simulink model "dtm"  (R2012b)
settings: Solver=ode45  StartTime=0.0  StopTime=15  RelTol=1e-3
settings Model: Creator=eechris  LastModifiedBy=eechris

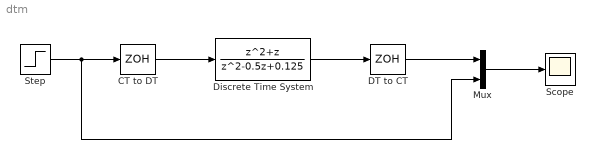
== system dtm ==
  CT to DT : ZeroOrderHold
  DT to CT : ZeroOrderHold
  Discrete Time System : DiscreteTransferFcn  Numerator=[1 1 0]  Denominator=[1 -0.5 0.125]
  Mux : Mux  Inputs=2
  Scope : Scope
      settings: YMin=0  YMax=4
  Step : Step  SampleTime=0
  wires:
  Step/1 -> Mux/2, CT to DT/1
  CT to DT/1 -> Discrete Time System/1
  Discrete Time System/1 -> DT to CT/1
  DT to CT/1 -> Mux/1
  Mux/1 -> Scope/1
